simulink model "DiscreteAutogen_Controller"  (R2022a)
settings: Solver=FixedStepAuto  StartTime=0.0  StopTime=TsimTime  FixedStep=Ts  MaxStep=Tsim*100  RelTol=1e-5
undefined symbols (not defined in the file): A, Arpm, Avdc, b, Brpm, Bvdc, DiscIntNeverNeededParam, IbuckSaturation, IsatLimit, K, Ki_d, Ki_q, Kiv, Kiw, Kp_d, Kp_q, Kpv, Kpw, Krpm, Ktv, Ld, Lq, P, Rdc, Ts
libraries: simulink x4
settings Model: Creator=MasterGnome  LastModifiedBy=MasterGnome
settings SolverCC: ZeroCrossAlgorithm=Adaptive
settings DataIOCC: SaveOutput=off  SaveTime=off
settings OptimizationCC: DefaultParameterBehavior=Inlined  EnhancedBackFolding=on  PassReuseOutputArgsAs=Individual arguments  ZeroExternalMemoryAtStartup=off  ZeroInternalMemoryAtStartup=off  OptimizeBlockOrder=speed  DifferentSizesBufferReuse=on  OptimizationCustomize=off  EfficientTunableParamExpr=on
settings DebuggingCC: IgnoredZcDiagnostic=none  ParameterTunabilityLossMsg=error  UnconnectedInputMsg=warning  UnconnectedOutputMsg=warning  UnconnectedLineMsg=warning
settings HardwareCC: ProdBitPerPointer=32  ProdBitPerSizeT=32  ProdBitPerPtrDiffT=32  ProdWordSize=32  ProdHWDeviceType=Intel->x86-32 (Windows32)  TargetBitPerPointer=64  TargetBitPerSizeT=64  TargetBitPerPtrDiffT=64  TargetLargestAtomicFloat=Float  TargetIntDivRoundTo=Zero  TargetEndianess=LittleEndian  TargetWordSize=64  TargetHWDeviceType=Intel->x86-64 (Windows64)
settings SFSimCC: MATLABDynamicMemAlloc=off
settings RTWCC: SystemTargetFile=ert.tlc  GenCodeOnly=on  TemplateMakefile=ert_default_tmf  DLArmComputeVersion=19.05
settings CodeAppCC: ForceParamTrailComments=on  IgnoreCustomStorageClasses=off  OperatorAnnotations=on  SimulinkDataObjDesc=on  SFDataObjDesc=on  InsertBlockDesc=on
settings ERTTargetCC: TargetLangStandard=C99 (ISO)  GenerateSampleERTMain=on  InlinedParameterPlacement=NonHierarchical  ERTCustomFileTemplate=example_file_process.tlc

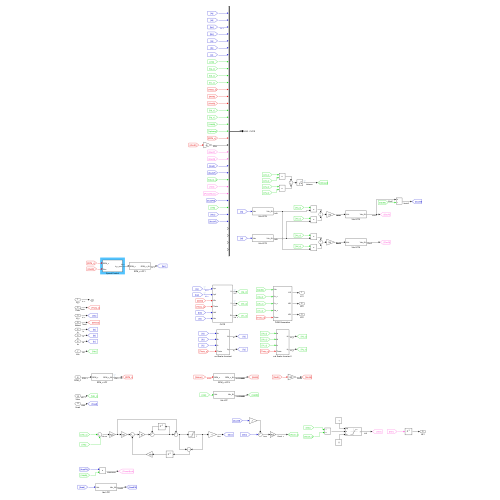
[thumbnail: Simulink's stored preview of the top-level diagram]
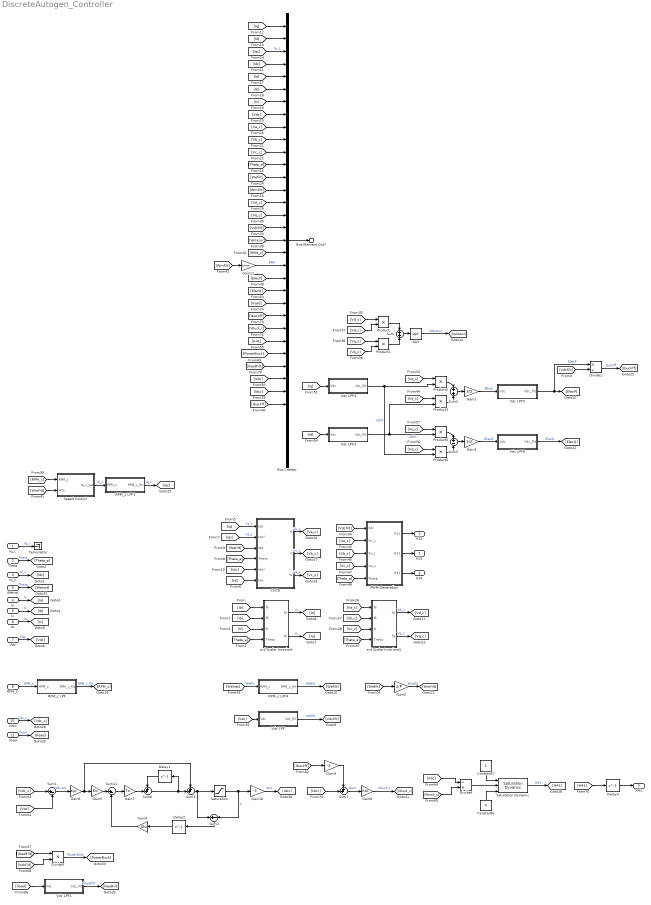
== system DiscreteAutogen_Controller ==
  Iq_c : Inport  OutDataTypeStr=double  PortDimensions=1
  Theta : Inport  Port=2  OutDataTypeStr=double  PortDimensions=1
  Id_c : Inport  Port=3  OutDataTypeStr=double  PortDimensions=1
  Iu : Inport  Port=4  OutDataTypeStr=double  PortDimensions=1
  Iv : Inport  Port=5  OutDataTypeStr=double  PortDimensions=1
  Iw : Inport  Port=6  OutDataTypeStr=double  PortDimensions=1
  Vdc : Inport  Port=7  OutDataTypeStr=double  PortDimensions=1
  RPM_C : Inport  Port=8  OutDataTypeStr=double  PortDimensions=1
  WeInst : Inport  Port=9  OutDataTypeStr=double  PortDimensions=1
  Vdcc : Inport  Port=10  OutDataTypeStr=double  PortDimensions=1
  Iload : Inport  Port=11  OutDataTypeStr=double  PortDimensions=1
  Bus Creator : BusCreator  Inputs=35
  CVCR : Subsystem
  Constant6 : Constant  Value=0
  Constant7 : Constant
  Delay1 : Delay  DelayLength=1  SampleTime=Ts
  Delay2 : Delay  DelayLength=1  SampleTime=Ts
  Delay3 : Delay  DelayLength=1  InitialCondition=0.1  SampleTime=Ts
  Divide1 : Product  Inputs=*/
  Divide3 : Product  Inputs=**
  Divide4 : Product  Inputs=/*
  Gain1 : Gain  Gain=3/2
  Gain11 : Gain  Gain=1/Krpm
  Gain16 : Gain  Gain=-1
  Gain2 : Gain  Gain=2/P
  Gain3 : Gain  Gain=3/2
  Gain4 : Gain  Gain=Ktv
  Gain5 : Gain  Gain=Kiv
  Gain6 : Gain  Gain=Kpv
  Gain7 : Gain  Gain=Ts
  Gain8 : Gain  Gain=Rdc
  Gain9 : Gain  Gain=-1
  PWM Generation : Subsystem
  Product{,1..3,5..6} (6 alike) : Product
  RPM_c LPF : Subsystem
  RPM_c LPF1 : Subsystem
  RPM_c LPF4 : Subsystem
  Saturation : Saturate  UpperLimit=0  LowerLimit=-IbuckSaturation
  Saturation Dynamic : simulink/Discontinuities/Saturation Dynamic  OutMin=[]  OutMax=[]  OutDataTypeStr=Inherit: Same as second input  OutDataType=fixdt(1, 16)  OutScaling=2^-10  DoSatur=off
  Speed Control : Subsystem
  Sqrt : Sqrt
  Sum : Sum  Inputs=+|+
  Sum1 : Sum  Inputs=|+-
  Sum11 : Sum  Inputs=|+-
  Sum2 : Sum  Inputs=+|+
  Sum3 : Sum  Inputs=++|
  Sum4 : Sum  Inputs=+|-
  Sum5 : Sum  Inputs=+|-
  Sum6 : Sum  Inputs=++|
  Sum7 : Sum  Inputs=++|
  Terminator : Terminator
  Vdc LPF : Subsystem
  Vdc LPF1 : Subsystem
  Vdc LPF3 : Subsystem
  Vdc LPF4 : Subsystem
  Vdc LPF5 : Subsystem
  Vdc LPF6 : Subsystem
  a-d Scalar Invariant : Subsystem
  a-d Scalar Invariant1 : Subsystem
  H11 : Outport  OutDataTypeStr=double  PortDimensions=1
  H21 : Outport  Port=2  OutDataTypeStr=double  PortDimensions=1
  H31 : Outport  Port=3  OutDataTypeStr=double  PortDimensions=1
  Bus Element Out7 : Outport  Port=4  PortName=LOG  Element=CVCR
  H41 : Outport  Port=5  OutDataTypeStr=double  PortDimensions=1
  wires:
  [Vc_c] -> PWM Generation/4(Vw_c)
  [Theta_e] -> PWM Generation/5(Theta)
  [Vb_c] -> PWM Generation/3(Vv_c)
  CVCR/2(V) -> [Vb_c]  "Vv_c"
  a-d Scalar Invariant/2(fq) -> [Iq]  "Iq"
  [Iq] -> CVCR/1(Iqe)  "Iq_c"
  CVCR/1(U) -> [Va_c]  "Vu_c"
  [Id] -> CVCR/6(Ide)
  CVCR/3(W) -> [Vc_c]  "Vw_c"
  [Vdcfilt] -> PWM Generation/1(Vdc)
  a-d Scalar Invariant/1(fd) -> [Id]  "Id"
  [Va_c] -> PWM Generation/2(Vu_c)
  PWM Generation/1(H11) -> H11/1
  PWM Generation/2(H21) -> H21/1
  PWM Generation/3(H31) -> H31/1
  [Wefilt] -> CVCR/3(We)
  [Theta_e] -> CVCR/4(Theta)
  [Theta_e] -> a-d Scalar Invariant/4(Theta)
  [Ib] -> a-d Scalar Invariant/2(fb)
  [Ic] -> a-d Scalar Invariant/3(fc)
  [Ia] -> a-d Scalar Invariant/1(fa)
  Iu/1 -> [Ia]  "Iu"
  Iv/1 -> [Ib]  "Iv"
  Iw/1 -> [Ic]  "Iw"
  Vdc/1 -> [Vdc]  "Vdc"
  [WeInst] -> RPM_c LPF4/1(RPM_c)  "Wefilt"
  Id_c/1 -> [Idc]  "Id_c"
  [Iqc] -> CVCR/2(Iqe*)  "Id_c"
  [Idc] -> CVCR/5(Ide*)
  Bus Creator/1 -> Bus Element Out7/1
  [Iq] -> Bus Creator/1
  [Id] -> Bus Creator/2
  [Iqc] -> Bus Creator/3  "Iq_c"
  [Idc] -> Bus Creator/4
  [Ia] -> Bus Creator/5
  [Ib] -> Bus Creator/6
  [Ic] -> Bus Creator/7
  [Vdc] -> Bus Creator/8
  [Va_c] -> Bus Creator/9
  [Vb_c] -> Bus Creator/10
  [Vc_c] -> Bus Creator/11
  [Theta_e] -> Bus Creator/12
  [Wefilt] -> Bus Creator/13
  [Theta_e] -> a-d Scalar Invariant1/4(Theta)
  [Va_c] -> a-d Scalar Invariant1/1(fa)
  [Vb_c] -> a-d Scalar Invariant1/2(fb)
  [Vc_c] -> a-d Scalar Invariant1/3(fc)
  a-d Scalar Invariant1/1(fd) -> [Vd_c]  "Vd_c"
  a-d Scalar Invariant1/2(fq) -> [Vq_c]  "Vq_c"
  [Vq_c] -> Bus Creator/16
  [Vd_c] -> Bus Creator/15
  [Wefilt] -> Gain2/1
  [Wmfilt] -> Bus Creator/14
  [Vdc] -> Vdc LPF/1(Vdc)
  Vdc LPF/1(Vdc_filt) -> [Vdcfilt]  "Vdcfilt"
  [Vdcfilt] -> Bus Creator/17
  [Vd_c] -> Product/1
  [Vd_c] -> Product/2
  [Vq_c] -> Product1/1
  [Vq_c] -> Product1/2
  Product/1 -> Sum/1
  Product1/1 -> Sum/2
  Sum/1 -> Sqrt/1
  Sqrt/1 -> [Vphasor]  "Vphasor"
  [Vphasor] -> Bus Creator/18
  Theta/1 -> [Theta_e]  "Theta"
  [Wmfilt] -> Speed Control/2(Wm)
  [RPM_c] -> Bus Creator/19
  Gain11/1 -> Bus Creator/20  "RPM"
  [Wmfilt] -> Gain11/1
  Speed Control/1(Iq_c_sat) -> RPM_c LPF1/1(RPM_c)  "Iq_c"
  [Vd_c] -> Product3/1
  Gain3/1 -> Vdc LPF6/1(Vdc)  "ElecQ"
  Product5/1 -> Sum5/1
  Sum2/1 -> Gain1/1
  Product3/1 -> Sum2/2
  Product2/1 -> Sum2/1
  Sum5/1 -> Gain3/1
  [Vq_c] -> Product2/1
  Product6/1 -> Sum5/2
  [Vd_c] -> Product6/1
  [Vq_c] -> Product5/1
  [ElecP] -> Bus Creator/21
  [ElecQ] -> Bus Creator/22
  RPM_C/1 -> RPM_c LPF/1(RPM_c)  "RPM_c"
  [RPM_c] -> Speed Control/1(RPM_c)
  RPM_c LPF/1(RPM_c_filt) -> [RPM_c]  "RPM_c_filt"
  Iq_c/1 -> Terminator/1  "Iq_c"
  RPM_c LPF1/1(RPM_c_filt) -> [Iqc]  "Iq_c"
  Gain2/1 -> [Wmfilt]  "Wmfilt"
  WeInst/1 -> [WeInst]  "Theta"
  RPM_c LPF4/1(RPM_c_filt) -> [Wefilt]  "Wefilt"
  Divide1/1 -> [Ibuckff]  "Ibuckff"
  Gain1/1 -> Vdc LPF5/1(Vdc)  "PElec"
  [Vdcfilt] -> Divide1/2
  Vdc LPF5/1(Vdc_filt) -> Divide1/1, [ElecP]  "ElecP"
  Vdc LPF6/1(Vdc_filt) -> [ElecQ]  "ElecQ"
  [Id] -> Vdc LPF3/1(Vdc)
  Vdc LPF3/1(Vdc_filt) -> Product3/2, Product5/2  "Idfilt"
  [Iq] -> Vdc LPF4/1(Vdc)
  Vdc LPF4/1(Vdc_filt) -> Product6/2, Product2/2  "Iqfilt"
  Sum4/1 -> Delay2/1
  [Vdcfilt] -> Divide3/2
  Delay2/1 -> Gain4/1
  Gain7/1 -> Sum6/2
  Vdc LPF1/1(Vdc_filt) -> [IloadFilt]  "Iloadfilt"
  Delay1/1 -> Sum6/1
  Gain16/1 -> [Idcc]  "Idcc"
  Sum6/1 -> Sum3/2, Delay1/1
  Constant6/1 -> Saturation Dynamic/3
  [Vbuck_c] -> Divide4/2
  Constant7/1 -> Saturation Dynamic/1
  [Vdc] -> Divide4/1
  [Vdc] -> Sum1/2
  Divide3/1 -> [PowerBuck]  "PowerBuck"
  [Iload] -> Vdc LPF1/1(Vdc)
  Saturation/1 -> Gain16/1, Sum4/2  "I*"
  [Vdc_c] -> Sum1/1
  Sum1/1 -> Gain6/1  "Vdc err"
  [H41] -> Delay3/1
  [Idcc] -> Sum7/2
  Sum7/1 -> Gain8/1  "Isum"
  Sum3/1 -> Sum4/1, Saturation/1
  Gain5/1 -> Sum11/1
  Divide4/1 -> Saturation Dynamic/2
  Sum11/1 -> Gain7/1
  Gain8/1 -> [Vbuck_c]  "Vbuck_c"
  [IloadFilt] -> Divide3/1
  Gain4/1 -> Sum11/2
  Vdcc/1 -> [Vdc_c]  "Vdc_c"
  Iload/1 -> [Iload]  "Iload"
  Saturation Dynamic/1 -> [H41]  "H41"
  Gain6/1 -> Gain5/1, Sum3/1
  [Vbuck_c] -> Bus Creator/25
  [Iload] -> Bus Creator/23
  [Ibuckff] -> Bus Creator/24
  [PowerBuck] -> Bus Creator/27
  [IloadFilt] -> Bus Creator/28
  [H41] -> Bus Creator/26
  [Ibuckff] -> Gain9/1
  Gain9/1 -> Sum7/1
  Delay3/1 -> H41/1
  [Vdc] -> Bus Creator/29
  [Idcc] -> Bus Creator/30
  [Ibuckff] -> Bus Creator/31

== system DiscreteAutogen_Controller/CVCR ==
  Iqe : Inport
  Iqe* : Inport  Port=2
  We : Inport  Port=3
  Theta : Inport  Port=4
  Ide* : Inport  Port=5
  Ide : Inport  Port=6
  "CVCR - Complex " : Subsystem  Commented=on
  CVCR Tustin Xcouple : Subsystem  Commented=on
  PI Tustin : Subsystem  Commented=on
  PI Zoh Parallel Xcouple : Subsystem  Commented=on
  PI Zoh Parallel1 : Subsystem  Commented=on
  PI Zoh Series : Subsystem  Commented=on
  PI Zoh Series Xcouple : Subsystem
  d-a Scalar Invariant : Subsystem
  q-a Scalar Invariant : Subsystem  Commented=on
  U : Outport
  V : Outport  Port=2
  W : Outport  Port=3
  wires:
  PI Zoh Series Xcouple/2(Vde) -> d-a Scalar Invariant/2(fd)  "Vd*"
  PI Zoh Series Xcouple/1(Vqe) -> d-a Scalar Invariant/1(fq)  "Vq*"
  Ide/1 -> PI Zoh Series Xcouple/5(Id)
  Ide*/1 -> PI Zoh Series Xcouple/4(Id_c)
  Iqe*/1 -> PI Zoh Series Xcouple/2(Iq_c)
  Iqe/1 -> PI Zoh Series Xcouple/1(Iq)
  d-a Scalar Invariant/2(b) -> V/1
  d-a Scalar Invariant/1(a) -> U/1
  Theta/1 -> d-a Scalar Invariant/3(theta)
  We/1 -> PI Zoh Series Xcouple/3(We)
  d-a Scalar Invariant/3(c) -> W/1

== system DiscreteAutogen_Controller/PWM Generation ==
  Vdc : Inport
  Vu_c : Inport  Port=2
  Vv_c : Inport  Port=3
  Vw_c : Inport  Port=4
  Theta : Inport  Port=5
  Duty Cycle Calc : Subsystem
  Modulation : Subsystem
  H11 : Outport
  H21 : Outport  Port=2
  H31 : Outport  Port=3
  wires:
  Vw_c/1 -> Modulation/4(Vc_c)
  Theta/1 -> Modulation/5(Theta)
  Vv_c/1 -> Modulation/3(Vb_c)
  Vu_c/1 -> Modulation/2(Va_c)
  Vdc/1 -> Modulation/1(Vdc), [Vdc]
  Duty Cycle Calc/3(H31) -> H31/1
  [Vdc] -> Duty Cycle Calc/1(Vdc)
  [Va_mod] -> Duty Cycle Calc/2(Va_mod)
  Modulation/3(Vc_mod) -> [Vc_mod]
  [Vc_mod] -> Duty Cycle Calc/4(Vc_mod)
  Duty Cycle Calc/2(H21) -> H21/1
  [Vb_mod] -> Duty Cycle Calc/3(Vb_mod)
  Duty Cycle Calc/1(H11) -> H11/1
  Modulation/2(Vb_mod) -> [Vb_mod]
  Modulation/1(Va_mod) -> [Va_mod]

== system DiscreteAutogen_Controller/RPM_c LPF ==
  RPM_c : Inport
  Delay2 : Delay  DelayLength=1  InitialCondition=0  SampleTime=Ts
  Gain1 : Gain  Gain=Brpm
  Gain3 : Gain  Gain=Arpm
  Sum2 : Sum  Inputs=|++
  RPM_c_filt : Outport
  wires:
  RPM_c/1 -> Gain1/1
  Delay2/1 -> RPM_c_filt/1, Gain3/1
  Sum2/1 -> Delay2/1
  Gain1/1 -> Sum2/1
  Gain3/1 -> Sum2/2

== system DiscreteAutogen_Controller/RPM_c LPF1 ==
  RPM_c : Inport
  Delay2 : Delay  DelayLength=1  InitialCondition=0  SampleTime=Ts
  Gain1 : Gain  Gain=Brpm
  Gain3 : Gain  Gain=Arpm
  Sum2 : Sum  Inputs=|++
  RPM_c_filt : Outport
  wires:
  RPM_c/1 -> Gain1/1
  Delay2/1 -> RPM_c_filt/1, Gain3/1
  Sum2/1 -> Delay2/1
  Gain1/1 -> Sum2/1
  Gain3/1 -> Sum2/2

== system DiscreteAutogen_Controller/RPM_c LPF4 ==
  RPM_c : Inport
  Delay2 : Delay  DelayLength=1  InitialCondition=0  SampleTime=Ts
  Gain1 : Gain  Gain=Brpm
  Gain3 : Gain  Gain=Arpm
  Sum2 : Sum  Inputs=|++
  RPM_c_filt : Outport
  wires:
  RPM_c/1 -> Gain1/1
  Delay2/1 -> RPM_c_filt/1, Gain3/1
  Sum2/1 -> Delay2/1
  Gain1/1 -> Sum2/1
  Gain3/1 -> Sum2/2

== system DiscreteAutogen_Controller/Speed Control ==
  RPM_c : Inport
  Wm : Inport  Port=2
  Delay1 : Delay  DelayLength=1  SampleTime=Ts
  Delay3 : Delay  DelayLength=1  SampleTime=Ts
  Gain11 : Gain  Gain=Krpm
  Gain4 : Gain  Gain=Kpw
  Gain5 : Gain  Gain=Ts
  Gain6 : Gain  Gain=Kiw
  Kt1 : Gain
  Saturation2 : Saturate  UpperLimit=IsatLimit  LowerLimit=-IsatLimit
  Sum11 : Sum  Inputs=+|-
  Sum12 : Sum  Inputs=|+-
  Sum6 : Sum  Inputs=++|
  Sum7 : Sum  Inputs=+++
  Sum9 : Sum  Inputs=|+-
  Iq_c_sat : Outport
  wires:
  Sum7/1 -> Saturation2/1, Sum11/1  "Iq_c_z"
  Sum12/1 -> Gain5/1
  Sum6/1 -> Sum7/2, Delay1/1
  Sum11/1 -> Delay3/1
  Sum9/1 -> Gain4/1
  Gain6/1 -> Sum12/1
  Gain5/1 -> Sum6/2
  Delay1/1 -> Sum6/1
  RPM_c/1 -> Gain11/1
  Gain11/1 -> Sum9/1  "Wm_c"
  Wm/1 -> Sum9/2
  Saturation2/1 -> Iq_c_sat/1, Sum11/2
  Delay3/1 -> Kt1/1
  Kt1/1 -> Sum12/2
  Gain4/1 -> Sum7/1, Gain6/1

== system DiscreteAutogen_Controller/Vdc LPF ==
  Vdc : Inport
  Delay2 : Delay  DelayLength=1  InitialCondition=0  SampleTime=Ts
  Gain1 : Gain  Gain=Bvdc
  Gain3 : Gain  Gain=Avdc
  Sum2 : Sum  Inputs=|++
  Vdc_filt : Outport
  wires:
  Vdc/1 -> Gain1/1
  Delay2/1 -> Vdc_filt/1, Gain3/1
  Sum2/1 -> Delay2/1
  Gain1/1 -> Sum2/1
  Gain3/1 -> Sum2/2

== system DiscreteAutogen_Controller/Vdc LPF1 ==
  Vdc : Inport
  Delay2 : Delay  DelayLength=1  InitialCondition=1  SampleTime=Ts
  Gain1 : Gain  Gain=Bvdc
  Gain3 : Gain  Gain=Avdc
  Sum2 : Sum  Inputs=|++
  Vdc_filt : Outport
  wires:
  Vdc/1 -> Gain1/1
  Delay2/1 -> Vdc_filt/1, Gain3/1
  Sum2/1 -> Delay2/1
  Gain1/1 -> Sum2/1
  Gain3/1 -> Sum2/2

== system DiscreteAutogen_Controller/Vdc LPF3 ==
  Vdc : Inport
  Delay2 : Delay  DelayLength=1  InitialCondition=0  SampleTime=Ts
  Gain1 : Gain  Gain=Bvdc
  Gain3 : Gain  Gain=Avdc
  Sum2 : Sum  Inputs=|++
  Vdc_filt : Outport
  wires:
  Vdc/1 -> Gain1/1
  Delay2/1 -> Vdc_filt/1, Gain3/1
  Sum2/1 -> Delay2/1
  Gain1/1 -> Sum2/1
  Gain3/1 -> Sum2/2

== system DiscreteAutogen_Controller/Vdc LPF4 ==
  Vdc : Inport
  Delay2 : Delay  DelayLength=1  InitialCondition=0  SampleTime=Ts
  Gain1 : Gain  Gain=Bvdc
  Gain3 : Gain  Gain=Avdc
  Sum2 : Sum  Inputs=|++
  Vdc_filt : Outport
  wires:
  Vdc/1 -> Gain1/1
  Delay2/1 -> Vdc_filt/1, Gain3/1
  Sum2/1 -> Delay2/1
  Gain1/1 -> Sum2/1
  Gain3/1 -> Sum2/2

== system DiscreteAutogen_Controller/Vdc LPF5 ==
  Vdc : Inport
  Delay2 : Delay  DelayLength=1  InitialCondition=0  SampleTime=Ts
  Gain1 : Gain  Gain=Bvdc
  Gain3 : Gain  Gain=Avdc
  Sum2 : Sum  Inputs=|++
  Vdc_filt : Outport
  wires:
  Vdc/1 -> Gain1/1
  Delay2/1 -> Vdc_filt/1, Gain3/1
  Sum2/1 -> Delay2/1
  Gain1/1 -> Sum2/1
  Gain3/1 -> Sum2/2

== system DiscreteAutogen_Controller/Vdc LPF6 ==
  Vdc : Inport
  Delay2 : Delay  DelayLength=1  InitialCondition=0  SampleTime=Ts
  Gain1 : Gain  Gain=Bvdc
  Gain3 : Gain  Gain=Avdc
  Sum2 : Sum  Inputs=|++
  Vdc_filt : Outport
  wires:
  Vdc/1 -> Gain1/1
  Delay2/1 -> Vdc_filt/1, Gain3/1
  Sum2/1 -> Delay2/1
  Gain1/1 -> Sum2/1
  Gain3/1 -> Sum2/2

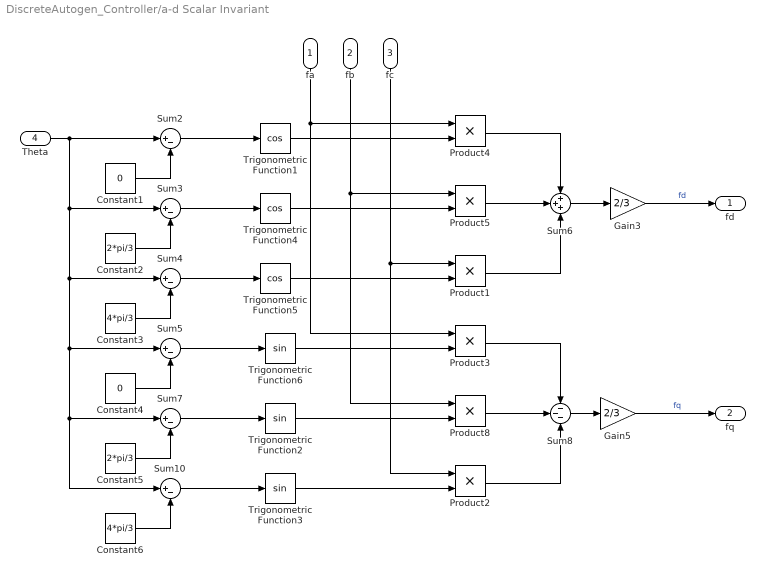
== system DiscreteAutogen_Controller/a-d Scalar Invariant ==
  fa : Inport
  fb : Inport  Port=2
  fc : Inport  Port=3
  Theta : Inport  Port=4
  Constant1 : Constant  Value=0
  Constant2 : Constant  Value=2*pi/3
  Constant3 : Constant  Value=4*pi/3
  Constant4 : Constant  Value=0
  Constant5 : Constant  Value=2*pi/3
  Constant6 : Constant  Value=4*pi/3
  Gain3 : Gain  Gain=2/3
  Gain5 : Gain  Gain=2/3
  Product{1..5,8} (6 alike) : Product
  Sum{2..5,7,10} (6 alike) : Sum  Inputs=|+-
  Sum6 : Sum  Inputs=+++
  Sum8 : Sum  Inputs=---
  Trigonometric Function1 : Trigonometry  Operator=cos
  Trigonometric Function2 : Trigonometry
  Trigonometric Function3 : Trigonometry
  Trigonometric Function4 : Trigonometry  Operator=cos
  Trigonometric Function5 : Trigonometry  Operator=cos
  Trigonometric Function6 : Trigonometry
  fd : Outport
  fq : Outport  Port=2
  wires:
  Product1/1 -> Sum6/3
  fc/1 -> Product2/1, Product1/1
  Sum4/1 -> Trigonometric Function5/1
  Constant5/1 -> Sum7/2
  Trigonometric Function4/1 -> Product5/2
  Sum7/1 -> Trigonometric Function2/1
  Constant6/1 -> Sum10/2
  Trigonometric Function3/1 -> Product2/2
  Theta/1 -> Sum10/1, Sum7/1, Sum5/1, Sum4/1, Sum3/1, Sum2/1
  Sum10/1 -> Trigonometric Function3/1
  Sum5/1 -> Trigonometric Function6/1
  Product2/1 -> Sum8/3
  Trigonometric Function2/1 -> Product8/2
  Product3/1 -> Sum8/1
  Constant3/1 -> Sum4/2
  Trigonometric Function1/1 -> Product4/2
  Product8/1 -> Sum8/2
  Trigonometric Function5/1 -> Product1/2
  Constant2/1 -> Sum3/2
  Sum3/1 -> Trigonometric Function4/1
  Sum8/1 -> Gain5/1
  Constant4/1 -> Sum5/2
  Constant1/1 -> Sum2/2
  Sum2/1 -> Trigonometric Function1/1
  fa/1 -> Product4/1, Product3/1
  Gain3/1 -> fd/1  "fd"
  Sum6/1 -> Gain3/1
  Trigonometric Function6/1 -> Product3/2
  Product4/1 -> Sum6/1
  Gain5/1 -> fq/1  "fq"
  fb/1 -> Product5/1, Product8/1
  Product5/1 -> Sum6/2

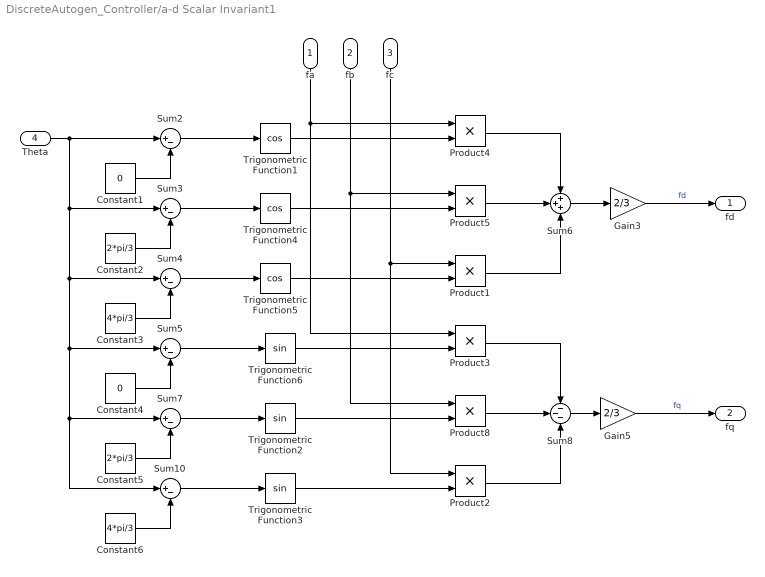
== system DiscreteAutogen_Controller/a-d Scalar Invariant1 ==
  fa : Inport
  fb : Inport  Port=2
  fc : Inport  Port=3
  Theta : Inport  Port=4
  Constant1 : Constant  Value=0
  Constant2 : Constant  Value=2*pi/3
  Constant3 : Constant  Value=4*pi/3
  Constant4 : Constant  Value=0
  Constant5 : Constant  Value=2*pi/3
  Constant6 : Constant  Value=4*pi/3
  Gain3 : Gain  Gain=2/3
  Gain5 : Gain  Gain=2/3
  Product{1..5,8} (6 alike) : Product
  Sum{2..5,7,10} (6 alike) : Sum  Inputs=|+-
  Sum6 : Sum  Inputs=+++
  Sum8 : Sum  Inputs=---
  Trigonometric Function1 : Trigonometry  Operator=cos
  Trigonometric Function2 : Trigonometry
  Trigonometric Function3 : Trigonometry
  Trigonometric Function4 : Trigonometry  Operator=cos
  Trigonometric Function5 : Trigonometry  Operator=cos
  Trigonometric Function6 : Trigonometry
  fd : Outport
  fq : Outport  Port=2
  wires:
  Product1/1 -> Sum6/3
  fc/1 -> Product2/1, Product1/1
  Sum4/1 -> Trigonometric Function5/1
  Constant5/1 -> Sum7/2
  Trigonometric Function4/1 -> Product5/2
  Sum7/1 -> Trigonometric Function2/1
  Constant6/1 -> Sum10/2
  Trigonometric Function3/1 -> Product2/2
  Theta/1 -> Sum10/1, Sum7/1, Sum5/1, Sum4/1, Sum3/1, Sum2/1
  Sum10/1 -> Trigonometric Function3/1
  Sum5/1 -> Trigonometric Function6/1
  Product2/1 -> Sum8/3
  Trigonometric Function2/1 -> Product8/2
  Product3/1 -> Sum8/1
  Constant3/1 -> Sum4/2
  Trigonometric Function1/1 -> Product4/2
  Product8/1 -> Sum8/2
  Trigonometric Function5/1 -> Product1/2
  Constant2/1 -> Sum3/2
  Sum3/1 -> Trigonometric Function4/1
  Sum8/1 -> Gain5/1
  Constant4/1 -> Sum5/2
  Constant1/1 -> Sum2/2
  Sum2/1 -> Trigonometric Function1/1
  fa/1 -> Product4/1, Product3/1
  Gain3/1 -> fd/1  "fd"
  Sum6/1 -> Gain3/1
  Trigonometric Function6/1 -> Product3/2
  Product4/1 -> Sum6/1
  Gain5/1 -> fq/1  "fq"
  fb/1 -> Product5/1, Product8/1
  Product5/1 -> Sum6/2

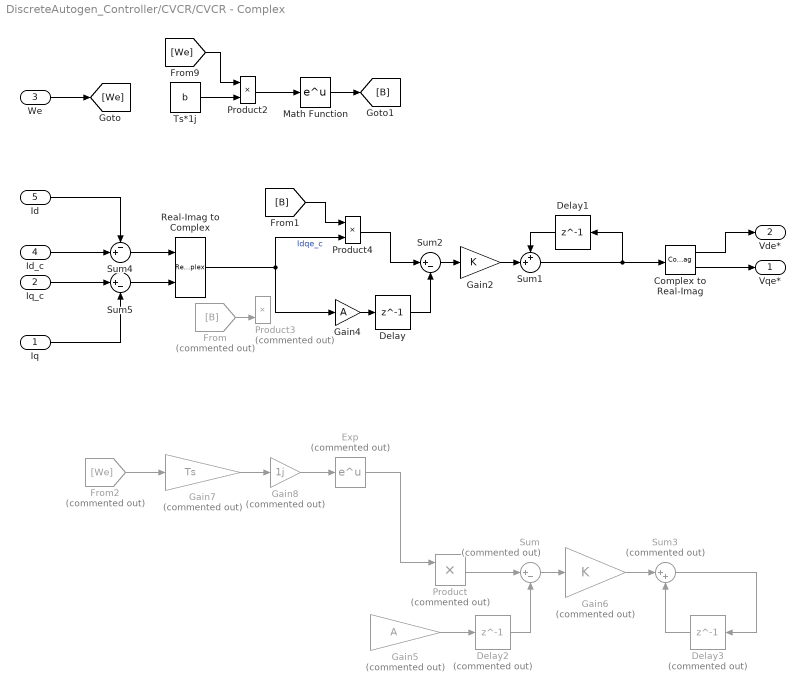
== system DiscreteAutogen_Controller/CVCR/CVCR - Complex  ==
  Iq : Inport
  Iq_c : Inport  Port=2
  We : Inport  Port=3
  Id_c : Inport  Port=4
  Id : Inport  Port=5
  Complex to Real-Imag : ComplexToRealImag
  Delay : Delay  DelayLength=1
  Delay1 : Delay  DelayLength=1
  Delay2 : Delay  Commented=on  DelayLength=1
  Delay3 : Delay  Commented=on  DelayLength=1
  Exp : Math  Commented=on
  From : From  Commented=on  GotoTag=B
  From2 : From  Commented=on  GotoTag=We
  Gain2 : Gain  Gain=K
  Gain4 : Gain  Gain=A
  Gain5 : Gain  Commented=on  Gain=A
  Gain6 : Gain  Commented=on  Gain=K
  Gain7 : Gain  Commented=on  Gain=Ts
  Gain8 : Gain  Commented=on  Gain=1j
  Math Function : Math
  Product : Product  Commented=on
  Product2 : Product
  Product3 : Product  Commented=on
  Product4 : Product
  Real-Imag to Complex : RealImagToComplex
  Sum : Sum  Commented=on  Inputs=|+-
  Sum1 : Sum  Inputs=++|
  Sum2 : Sum  Inputs=|+-
  Sum3 : Sum  Commented=on  Inputs=|++
  Sum4 : Sum  Inputs=-+|
  Sum5 : Sum  Inputs=|+-
  Ts*1j : Constant  Value=b
  Vqe* : Outport
  Vde* : Outport  Port=2
  wires:
  Sum5/1 -> Real-Imag to Complex/2
  Sum4/1 -> Real-Imag to Complex/1
  Id_c/1 -> Sum4/2
  Id/1 -> Sum4/1
  Iq_c/1 -> Sum5/1
  Iq/1 -> Sum5/2
  Complex to Real-Imag/2 -> Vqe*/1
  Complex to Real-Imag/1 -> Vde*/1
  We/1 -> [We]
  [We] -> Product2/1
  Math Function/1 -> [B]
  From/1 -> Product3/2
  Gain4/1 -> Delay/1
  Delay/1 -> Sum2/2
  Delay1/1 -> Sum1/1
  Product2/1 -> Math Function/1
  Sum2/1 -> Gain2/1
  Gain2/1 -> Sum1/2
  Sum1/1 -> Complex to Real-Imag/1, Delay1/1
  [B] -> Product4/1
  Product4/1 -> Sum2/1
  From2/1 -> Gain7/1
  Sum/1 -> Gain6/1
  Sum3/1 -> Delay3/1
  Gain5/1 -> Delay2/1
  Exp/1 -> Product/1
  Delay2/1 -> Sum/2
  Gain6/1 -> Sum3/1
  Delay3/1 -> Sum3/2
  Product/1 -> Sum/1
  Gain7/1 -> Gain8/1
  Gain8/1 -> Exp/1
  ? -> Gain5/1, Product/2
  Ts*1j/1 -> Product2/2
  Real-Imag to Complex/1 -> Product4/2, Gain4/1  "Idqe_c"

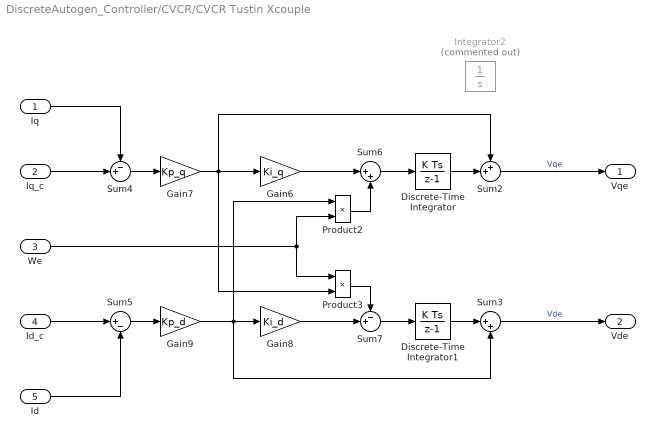
== system DiscreteAutogen_Controller/CVCR/CVCR Tustin Xcouple ==
  Iq : Inport
  Iq_c : Inport  Port=2
  We : Inport  Port=3
  Id_c : Inport  Port=4
  Id : Inport  Port=5
  Discrete-Time Integrator : DiscreteIntegrator  SampleTime=Ts  ICPrevOutput=DiscIntNeverNeededParam  ICPrevScaledInput=DiscIntNeverNeededParam
  Discrete-Time Integrator1 : DiscreteIntegrator  SampleTime=Ts  ICPrevOutput=DiscIntNeverNeededParam  ICPrevScaledInput=DiscIntNeverNeededParam
  Gain6 : Gain  Gain=Ki_q
  Gain7 : Gain  Gain=Kp_q
  Gain8 : Gain  Gain=Ki_d
  Gain9 : Gain  Gain=Kp_d
  Integrator2 : Integrator  Commented=on
  Product2 : Product
  Product3 : Product
  Sum2 : Sum  Inputs=++|
  Sum3 : Sum  Inputs=|++
  Sum4 : Sum  Inputs=-+|
  Sum5 : Sum  Inputs=|+-
  Sum6 : Sum  Inputs=|++
  Sum7 : Sum  Inputs=-+|
  Vqe : Outport
  Vde : Outport  Port=2
  wires:
  Sum3/1 -> Vde/1  "Vde"
  Id_c/1 -> Sum5/1
  Sum2/1 -> Vqe/1  "Vqe"
  Iq/1 -> Sum4/1
  Gain6/1 -> Sum6/1
  Sum7/1 -> Discrete-Time Integrator1/1
  Sum4/1 -> Gain7/1
  Gain8/1 -> Sum7/2
  Discrete-Time Integrator/1 -> Sum2/2
  Iq_c/1 -> Sum4/2
  Id/1 -> Sum5/2
  Sum6/1 -> Discrete-Time Integrator/1
  Product3/1 -> Sum7/1
  Gain7/1 -> Product3/2, Sum2/1, Gain6/1
  Product2/1 -> Sum6/2
  Discrete-Time Integrator1/1 -> Sum3/1
  Sum5/1 -> Gain9/1
  Gain9/1 -> Sum3/2, Gain8/1, Product2/1
  We/1 -> Product3/1, Product2/2

== system DiscreteAutogen_Controller/CVCR/PI Tustin ==
  Iq : Inport
  Iq_c : Inport  Port=2
  We : Inport  Port=3
  Id_c : Inport  Port=4
  Id : Inport  Port=5
  Discrete-Time Integrator : DiscreteIntegrator  SampleTime=Ts  ICPrevOutput=DiscIntNeverNeededParam  ICPrevScaledInput=DiscIntNeverNeededParam
  Discrete-Time Integrator1 : DiscreteIntegrator  SampleTime=Ts  ICPrevOutput=DiscIntNeverNeededParam  ICPrevScaledInput=DiscIntNeverNeededParam
  Gain6 : Gain  Gain=Ki_q
  Gain7 : Gain  Gain=Kp_q
  Gain8 : Gain  Gain=Ki_d
  Gain9 : Gain  Gain=Kp_d
  Sum2 : Sum  Inputs=++|
  Sum3 : Sum  Inputs=|++
  Sum4 : Sum  Inputs=-+|
  Sum5 : Sum  Inputs=|+-
  Sum6 : Sum  Inputs=|++
  Sum7 : Sum  Inputs=-+|
  Vqe : Outport
  Vde : Outport  Port=2
  wires:
  Sum3/1 -> Vde/1  "Vde"
  Id_c/1 -> Sum5/1
  Sum2/1 -> Vqe/1  "Vqe"
  Iq/1 -> Sum4/1
  Gain6/1 -> Sum6/1
  Sum7/1 -> Discrete-Time Integrator1/1
  Sum4/1 -> Gain7/1
  Gain8/1 -> Sum7/2
  Discrete-Time Integrator/1 -> Sum2/2
  Iq_c/1 -> Sum4/2
  Id/1 -> Sum5/2
  Sum6/1 -> Discrete-Time Integrator/1
  Gain7/1 -> Sum2/1, Gain6/1
  Discrete-Time Integrator1/1 -> Sum3/1
  Sum5/1 -> Gain9/1
  Gain9/1 -> Sum3/2, Gain8/1

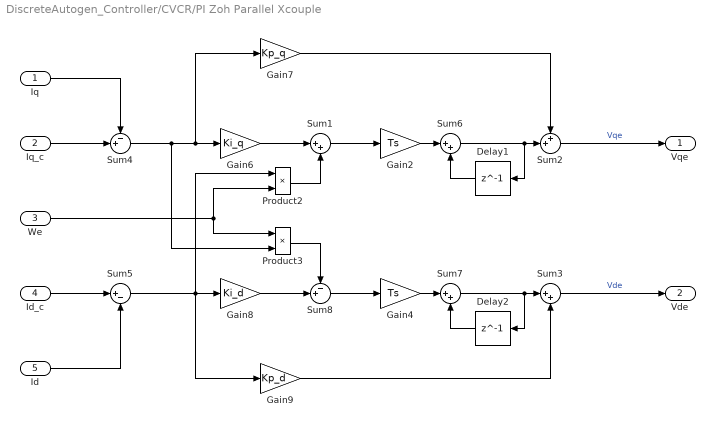
== system DiscreteAutogen_Controller/CVCR/PI Zoh Parallel Xcouple ==
  Iq : Inport
  Iq_c : Inport  Port=2
  We : Inport  Port=3
  Id_c : Inport  Port=4
  Id : Inport  Port=5
  Delay1 : Delay  DelayLength=1  SampleTime=Ts
  Delay2 : Delay  DelayLength=1  SampleTime=Ts
  Gain2 : Gain  Gain=Ts
  Gain4 : Gain  Gain=Ts
  Gain6 : Gain  Gain=Ki_q
  Gain7 : Gain  Gain=Kp_q
  Gain8 : Gain  Gain=Ki_d
  Gain9 : Gain  Gain=Kp_d
  Product2 : Product
  Product3 : Product
  Sum{1,3,6..7} (4 alike) : Sum  Inputs=|++
  Sum2 : Sum  Inputs=++|
  Sum4 : Sum  Inputs=-+|
  Sum5 : Sum  Inputs=|+-
  Sum8 : Sum  Inputs=-+|
  Vqe : Outport
  Vde : Outport  Port=2
  wires:
  Sum3/1 -> Vde/1  "Vde"
  Id_c/1 -> Sum5/1
  Sum2/1 -> Vqe/1  "Vqe"
  Iq/1 -> Sum4/1
  Gain6/1 -> Sum1/1
  Sum6/1 -> Delay1/1, Sum2/2
  Iq_c/1 -> Sum4/2
  Id/1 -> Sum5/2
  Gain7/1 -> Sum2/1
  Gain9/1 -> Sum3/2
  Gain2/1 -> Sum6/1
  Delay1/1 -> Sum6/2
  Gain4/1 -> Sum7/1
  Delay2/1 -> Sum7/2
  Sum7/1 -> Sum3/1, Delay2/1
  Sum4/1 -> Product3/2, Gain6/1, Gain7/1
  Product3/1 -> Sum8/1
  Sum5/1 -> Gain9/1, Product2/1, Gain8/1
  Product2/1 -> Sum1/2
  We/1 -> Product3/1, Product2/2
  Sum1/1 -> Gain2/1
  Gain8/1 -> Sum8/2
  Sum8/1 -> Gain4/1

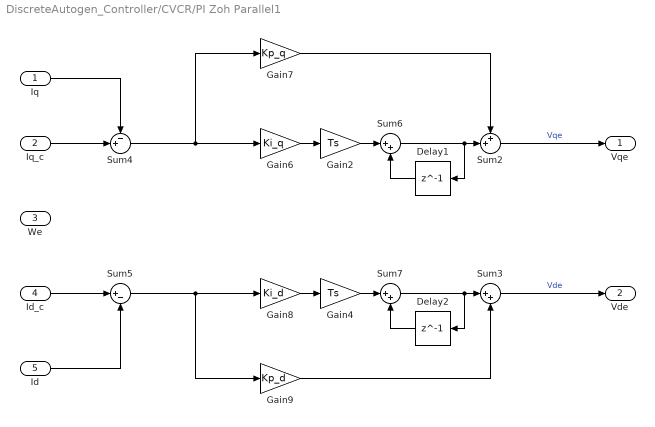
== system DiscreteAutogen_Controller/CVCR/PI Zoh Parallel1 ==
  Iq : Inport
  Iq_c : Inport  Port=2
  We : Inport  Port=3
  Id_c : Inport  Port=4
  Id : Inport  Port=5
  Delay1 : Delay  DelayLength=1  SampleTime=Ts
  Delay2 : Delay  DelayLength=1  SampleTime=Ts
  Gain2 : Gain  Gain=Ts
  Gain4 : Gain  Gain=Ts
  Gain6 : Gain  Gain=Ki_q
  Gain7 : Gain  Gain=Kp_q
  Gain8 : Gain  Gain=Ki_d
  Gain9 : Gain  Gain=Kp_d
  Sum2 : Sum  Inputs=++|
  Sum3 : Sum  Inputs=|++
  Sum4 : Sum  Inputs=-+|
  Sum5 : Sum  Inputs=|+-
  Sum6 : Sum  Inputs=|++
  Sum7 : Sum  Inputs=|++
  Vqe : Outport
  Vde : Outport  Port=2
  wires:
  Sum3/1 -> Vde/1  "Vde"
  Id_c/1 -> Sum5/1
  Sum2/1 -> Vqe/1  "Vqe"
  Iq/1 -> Sum4/1
  Gain6/1 -> Gain2/1
  Sum4/1 -> Gain6/1, Gain7/1
  Sum6/1 -> Delay1/1, Sum2/2
  Iq_c/1 -> Sum4/2
  Id/1 -> Sum5/2
  Gain7/1 -> Sum2/1
  Sum5/1 -> Gain8/1, Gain9/1
  Gain9/1 -> Sum3/2
  Gain2/1 -> Sum6/1
  Delay1/1 -> Sum6/2
  Gain4/1 -> Sum7/1
  Delay2/1 -> Sum7/2
  Sum7/1 -> Sum3/1, Delay2/1
  Gain8/1 -> Gain4/1

== system DiscreteAutogen_Controller/CVCR/PI Zoh Series ==
  Iq : Inport
  Iq_c : Inport  Port=2
  We : Inport  Port=3
  Id_c : Inport  Port=4
  Id : Inport  Port=5
  Delay1 : Delay  DelayLength=1  SampleTime=Ts
  Delay2 : Delay  DelayLength=1  SampleTime=Ts
  Gain2 : Gain  Gain=Ts
  Gain4 : Gain  Gain=Ts
  Gain6 : Gain  Gain=Ki_q
  Gain7 : Gain  Gain=Kp_q
  Gain8 : Gain  Gain=Ki_d
  Gain9 : Gain  Gain=Kp_d
  Sum2 : Sum  Inputs=++|
  Sum3 : Sum  Inputs=|++
  Sum4 : Sum  Inputs=-+|
  Sum5 : Sum  Inputs=|+-
  Sum6 : Sum  Inputs=|++
  Sum7 : Sum  Inputs=|++
  Vqe : Outport
  Vde : Outport  Port=2
  wires:
  Sum3/1 -> Vde/1  "Vde"
  Id_c/1 -> Sum5/1
  Sum2/1 -> Vqe/1  "Vqe"
  Iq/1 -> Sum4/1
  Gain6/1 -> Gain2/1
  Sum4/1 -> Gain7/1
  Sum6/1 -> Delay1/1, Sum2/2
  Iq_c/1 -> Sum4/2
  Id/1 -> Sum5/2
  Gain7/1 -> Sum2/1, Gain6/1
  Sum5/1 -> Gain9/1
  Gain9/1 -> Sum3/2, Gain8/1
  Gain2/1 -> Sum6/1
  Delay1/1 -> Sum6/2
  Gain4/1 -> Sum7/1
  Delay2/1 -> Sum7/2
  Sum7/1 -> Sum3/1, Delay2/1
  Gain8/1 -> Gain4/1

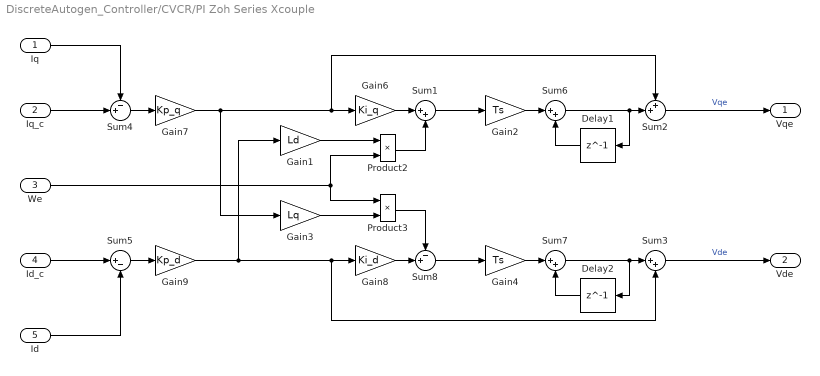
== system DiscreteAutogen_Controller/CVCR/PI Zoh Series Xcouple ==
  Iq : Inport
  Iq_c : Inport  Port=2
  We : Inport  Port=3
  Id_c : Inport  Port=4
  Id : Inport  Port=5
  Delay1 : Delay  DelayLength=1  SampleTime=Ts
  Delay2 : Delay  DelayLength=1  SampleTime=Ts
  Gain1 : Gain  Gain=Ld
  Gain2 : Gain  Gain=Ts
  Gain3 : Gain  Gain=Lq
  Gain4 : Gain  Gain=Ts
  Gain6 : Gain  Gain=Ki_q
  Gain7 : Gain  Gain=Kp_q
  Gain8 : Gain  Gain=Ki_d
  Gain9 : Gain  Gain=Kp_d
  Product2 : Product
  Product3 : Product
  Sum{1,3,6..7} (4 alike) : Sum  Inputs=|++
  Sum2 : Sum  Inputs=++|
  Sum4 : Sum  Inputs=-+|
  Sum5 : Sum  Inputs=|+-
  Sum8 : Sum  Inputs=-+|
  Vqe : Outport
  Vde : Outport  Port=2
  wires:
  Sum3/1 -> Vde/1  "Vde"
  Id_c/1 -> Sum5/1
  Sum2/1 -> Vqe/1  "Vqe"
  Iq/1 -> Sum4/1
  Gain6/1 -> Sum1/1
  Sum6/1 -> Delay1/1, Sum2/2
  Iq_c/1 -> Sum4/2
  Id/1 -> Sum5/2
  Gain7/1 -> Gain3/1, Sum2/1, Gain6/1
  Gain9/1 -> Gain1/1, Sum3/2, Gain8/1
  Gain2/1 -> Sum6/1
  Delay1/1 -> Sum6/2
  Gain4/1 -> Sum7/1
  Delay2/1 -> Sum7/2
  Sum7/1 -> Sum3/1, Delay2/1
  Sum4/1 -> Gain7/1
  Product3/1 -> Sum8/1
  Sum5/1 -> Gain9/1
  Product2/1 -> Sum1/2
  Sum1/1 -> Gain2/1
  Gain8/1 -> Sum8/2
  Sum8/1 -> Gain4/1
  We/1 -> Product2/2, Product3/1
  Gain1/1 -> Product2/1
  Gain3/1 -> Product3/2

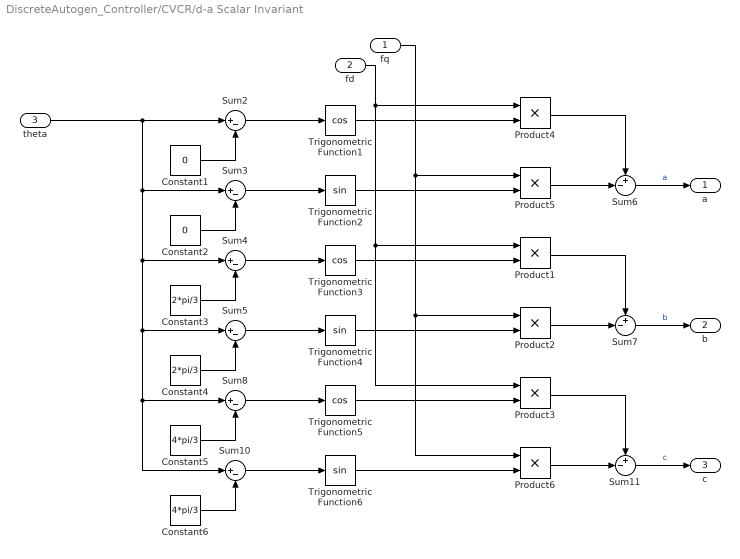
== system DiscreteAutogen_Controller/CVCR/d-a Scalar Invariant ==
  fq : Inport
  fd : Inport  Port=2
  theta : Inport  Port=3
  Constant1 : Constant  Value=0
  Constant2 : Constant  Value=0
  Constant3 : Constant  Value=2*pi/3
  Constant4 : Constant  Value=2*pi/3
  Constant5 : Constant  Value=4*pi/3
  Constant6 : Constant  Value=4*pi/3
  Product{1..6} (6 alike) : Product
  Sum{2..5,8,10} (6 alike) : Sum  Inputs=|+-
  Sum11 : Sum  Inputs=+-|
  Sum6 : Sum  Inputs=+-|
  Sum7 : Sum  Inputs=+-|
  Trigonometric Function1 : Trigonometry  Operator=cos
  Trigonometric Function2 : Trigonometry
  Trigonometric Function3 : Trigonometry  Operator=cos
  Trigonometric Function4 : Trigonometry
  Trigonometric Function5 : Trigonometry  Operator=cos
  Trigonometric Function6 : Trigonometry
  a : Outport
  b : Outport  Port=2
  c : Outport  Port=3
  wires:
  theta/1 -> Sum2/1, Sum3/1, Sum4/1, Sum5/1, Sum8/1, Sum10/1
  Trigonometric Function6/1 -> Product6/2
  Trigonometric Function5/1 -> Product3/2
  Constant4/1 -> Sum5/2
  Product1/1 -> Sum7/1
  Trigonometric Function1/1 -> Product4/2
  Product6/1 -> Sum11/2
  Sum10/1 -> Trigonometric Function6/1
  fd/1 -> Product3/1, Product1/1, Product4/1
  Sum3/1 -> Trigonometric Function2/1
  fq/1 -> Product6/1, Product2/1, Product5/1
  Product5/1 -> Sum6/2
  Trigonometric Function2/1 -> Product5/2
  Constant6/1 -> Sum10/2
  Sum8/1 -> Trigonometric Function5/1
  Sum2/1 -> Trigonometric Function1/1
  Sum4/1 -> Trigonometric Function3/1
  Constant1/1 -> Sum2/2
  Product2/1 -> Sum7/2
  Trigonometric Function3/1 -> Product1/2
  Sum5/1 -> Trigonometric Function4/1
  Trigonometric Function4/1 -> Product2/2
  Constant5/1 -> Sum8/2
  Sum6/1 -> a/1  "a"
  Constant3/1 -> Sum4/2
  Product3/1 -> Sum11/1
  Product4/1 -> Sum6/1
  Constant2/1 -> Sum3/2
  Sum11/1 -> c/1  "c"
  Sum7/1 -> b/1  "b"

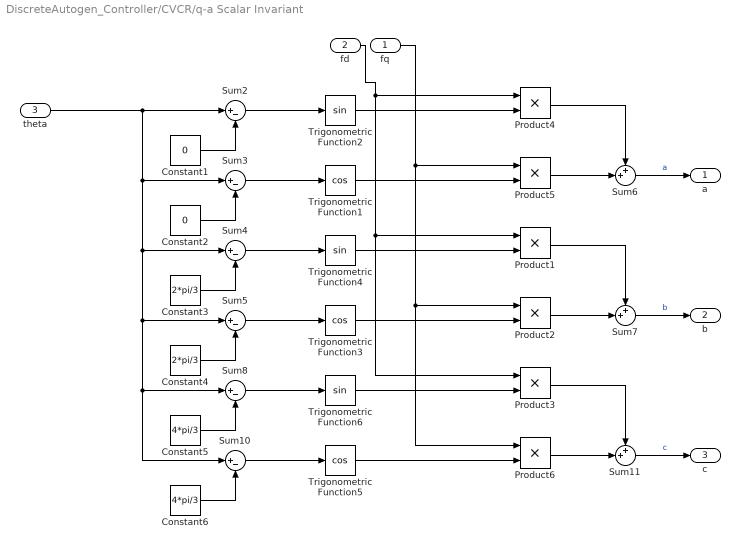
== system DiscreteAutogen_Controller/CVCR/q-a Scalar Invariant ==
  fq : Inport
  fd : Inport  Port=2
  theta : Inport  Port=3
  Constant1 : Constant  Value=0
  Constant2 : Constant  Value=0
  Constant3 : Constant  Value=2*pi/3
  Constant4 : Constant  Value=2*pi/3
  Constant5 : Constant  Value=4*pi/3
  Constant6 : Constant  Value=4*pi/3
  Product{1..6} (6 alike) : Product
  Sum{2..5,8,10} (6 alike) : Sum  Inputs=|+-
  Sum11 : Sum  Inputs=++|
  Sum6 : Sum  Inputs=++|
  Sum7 : Sum  Inputs=++|
  Trigonometric Function1 : Trigonometry  Operator=cos
  Trigonometric Function2 : Trigonometry
  Trigonometric Function3 : Trigonometry  Operator=cos
  Trigonometric Function4 : Trigonometry
  Trigonometric Function5 : Trigonometry  Operator=cos
  Trigonometric Function6 : Trigonometry
  a : Outport
  b : Outport  Port=2
  c : Outport  Port=3
  wires:
  Sum7/1 -> b/1  "b"
  Sum11/1 -> c/1  "c"
  Constant2/1 -> Sum3/2
  Product4/1 -> Sum6/1
  Product3/1 -> Sum11/1
  Constant3/1 -> Sum4/2
  Sum6/1 -> a/1  "a"
  Constant5/1 -> Sum8/2
  Trigonometric Function3/1 -> Product2/2
  Sum5/1 -> Trigonometric Function3/1
  Trigonometric Function4/1 -> Product1/2
  Product2/1 -> Sum7/2
  Constant1/1 -> Sum2/2
  Sum4/1 -> Trigonometric Function4/1
  Sum2/1 -> Trigonometric Function2/1
  Sum8/1 -> Trigonometric Function6/1
  Constant6/1 -> Sum10/2
  Trigonometric Function1/1 -> Product5/2
  Product5/1 -> Sum6/2
  fq/1 -> Product5/1, Product2/1, Product6/1
  Sum3/1 -> Trigonometric Function1/1
  fd/1 -> Product4/1, Product1/1, Product3/1
  Sum10/1 -> Trigonometric Function5/1
  Product6/1 -> Sum11/2
  Trigonometric Function2/1 -> Product4/2
  Product1/1 -> Sum7/1
  Constant4/1 -> Sum5/2
  Trigonometric Function6/1 -> Product3/2
  Trigonometric Function5/1 -> Product6/2
  theta/1 -> Sum10/1, Sum8/1, Sum5/1, Sum4/1, Sum3/1, Sum2/1

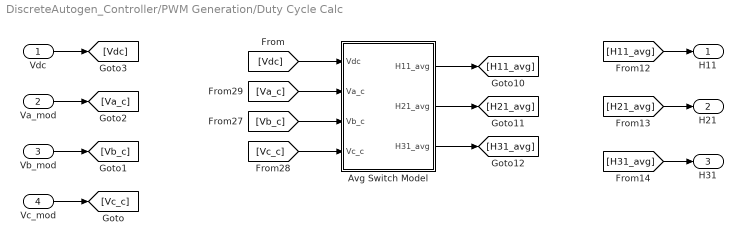
== system DiscreteAutogen_Controller/PWM Generation/Duty Cycle Calc ==
  Vdc : Inport
  Va_mod : Inport  Port=2
  Vb_mod : Inport  Port=3
  Vc_mod : Inport  Port=4
  Avg Switch Model : Subsystem
  H11 : Outport
  H21 : Outport  Port=2
  H31 : Outport  Port=3
  wires:
  Vdc/1 -> [Vdc]
  Vb_mod/1 -> [Vb_c]
  Va_mod/1 -> [Va_c]
  Vc_mod/1 -> [Vc_c]
  Avg Switch Model/3(H31_avg) -> [H31_avg]
  Avg Switch Model/2(H21_avg) -> [H21_avg]
  Avg Switch Model/1(H11_avg) -> [H11_avg]
  [Vc_c] -> Avg Switch Model/4(Vc_c)
  [Vb_c] -> Avg Switch Model/3(Vb_c)
  [Va_c] -> Avg Switch Model/2(Va_c)
  [Vdc] -> Avg Switch Model/1(Vdc)
  [H11_avg] -> H11/1
  [H21_avg] -> H21/1
  [H31_avg] -> H31/1

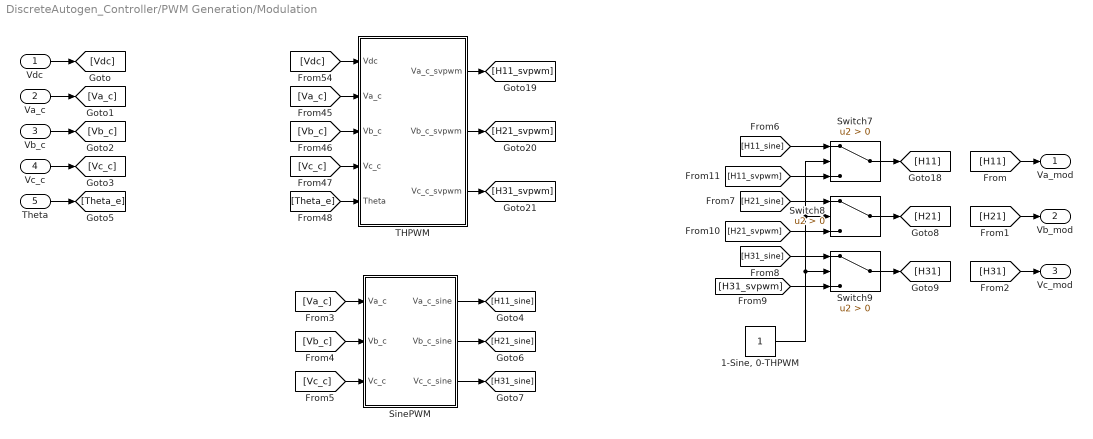
== system DiscreteAutogen_Controller/PWM Generation/Modulation ==
  Vdc : Inport
  Va_c : Inport  Port=2
  Vb_c : Inport  Port=3
  Vc_c : Inport  Port=4
  Theta : Inport  Port=5
  "1-Sine, 0-THPWM" : Constant
  SinePWM : Subsystem
  Switch7 : Switch  Criteria=u2 > Threshold  ZeroCross=off  SaturateOnIntegerOverflow=off  InputSameDT=off
  Switch8 : Switch  Criteria=u2 > Threshold  ZeroCross=off  SaturateOnIntegerOverflow=off  InputSameDT=off
  Switch9 : Switch  Criteria=u2 > Threshold  ZeroCross=off  SaturateOnIntegerOverflow=off  InputSameDT=off
  THPWM : Subsystem
  Va_mod : Outport
  Vb_mod : Outport  Port=2
  Vc_mod : Outport  Port=3
  wires:
  [Vc_c] -> SinePWM/3(Vc_c)
  [Va_c] -> SinePWM/1(Va_c)
  [Vb_c] -> SinePWM/2(Vb_c)
  SinePWM/3(Vc_c_sine) -> [H31_sine]
  SinePWM/2(Vb_c_sine) -> [H21_sine]
  SinePWM/1(Va_c_sine) -> [H11_sine]
  Switch8/1 -> [H21]
  [H31_sine] -> Switch9/1
  "1-Sine, 0-THPWM"/1 -> Switch7/2, Switch8/2, Switch9/2
  [H31_svpwm] -> Switch9/3
  Switch7/1 -> [H11]
  [H11_sine] -> Switch7/1
  [H21_svpwm] -> Switch8/3
  [H11_svpwm] -> Switch7/3
  Switch9/1 -> [H31]
  [H21_sine] -> Switch8/1
  [H31] -> Vc_mod/1
  [H21] -> Vb_mod/1
  [H11] -> Va_mod/1
  THPWM/3(Vc_c_svpwm) -> [H31_svpwm]
  THPWM/2(Vb_c_svpwm) -> [H21_svpwm]
  THPWM/1(Va_c_svpwm) -> [H11_svpwm]
  [Theta_e] -> THPWM/5(Theta)
  [Vc_c] -> THPWM/4(Vc_c)
  [Vb_c] -> THPWM/3(Vb_c)
  [Va_c] -> THPWM/2(Va_c)
  [Vdc] -> THPWM/1(Vdc)
  Theta/1 -> [Theta_e]
  Vc_c/1 -> [Vc_c]
  Vb_c/1 -> [Vb_c]
  Va_c/1 -> [Va_c]
  Vdc/1 -> [Vdc]

== system DiscreteAutogen_Controller/PWM Generation/Duty Cycle Calc/Avg Switch Model ==
  Vdc : Inport
  Va_c : Inport  Port=2
  Vb_c : Inport  Port=3
  Vc_c : Inport  Port=4
  Constant2 : Constant  Value=2
  Constant6 : Constant  Value=0
  Constant7 : Constant
  Divide{4..7} (4 alike) : Product  Inputs=/*
  Saturation Dynamic : simulink/Discontinuities/Saturation Dynamic  OutMin=[]  OutMax=[]  OutDataTypeStr=Inherit: Same as second input  OutDataType=fixdt(1, 16)  OutScaling=2^-10  DoSatur=off
  Saturation Dynamic1 : simulink/Discontinuities/Saturation Dynamic  OutMin=[]  OutMax=[]  OutDataTypeStr=Inherit: Same as second input  OutDataType=fixdt(1, 16)  OutScaling=2^-10  DoSatur=off
  Saturation Dynamic2 : simulink/Discontinuities/Saturation Dynamic  OutMin=[]  OutMax=[]  OutDataTypeStr=Inherit: Same as second input  OutDataType=fixdt(1, 16)  OutScaling=2^-10  DoSatur=off
  Sum1 : Sum  Inputs=++|
  Sum4 : Sum  Inputs=++|
  Sum5 : Sum  Inputs=++|
  H11_avg : Outport
  H21_avg : Outport  Port=2
  H31_avg : Outport  Port=3
  wires:
  Saturation Dynamic1/1 -> H21_avg/1
  Saturation Dynamic/1 -> H11_avg/1
  Vb_c/1 -> Sum4/2
  Vc_c/1 -> Sum1/2
  Vdc/1 -> Divide5/2, Divide4/1, Divide6/1, Divide7/1
  Va_c/1 -> Sum5/2
  Sum5/1 -> Divide4/2
  Divide7/1 -> Saturation Dynamic2/2
  Saturation Dynamic2/1 -> H31_avg/1
  Sum1/1 -> Divide7/2
  Divide6/1 -> Saturation Dynamic1/2
  Divide4/1 -> Saturation Dynamic/2
  Sum4/1 -> Divide6/2
  Constant6/1 -> Saturation Dynamic/3, Saturation Dynamic1/3, Saturation Dynamic2/3
  Constant2/1 -> Divide5/1
  Constant7/1 -> Saturation Dynamic2/1, Saturation Dynamic1/1, Saturation Dynamic/1
  Divide5/1 -> Sum5/1, Sum4/1, Sum1/1

== system DiscreteAutogen_Controller/PWM Generation/Modulation/SinePWM ==
  Va_c : Inport
  Vb_c : Inport  Port=2
  Vc_c : Inport  Port=3
  Va_c_sine : Outport
  Vb_c_sine : Outport  Port=2
  Vc_c_sine : Outport  Port=3
  wires:
  [H31_sine] -> Vc_c_sine/1
  [H21_sine] -> Vb_c_sine/1
  Vc_c/1 -> [Vc_c]
  Vb_c/1 -> [Vb_c]
  [H11_sine] -> Va_c_sine/1
  Va_c/1 -> [Va_c]
  [Va_c] -> [H11_sine]
  [Vb_c] -> [H21_sine]
  [Vc_c] -> [H31_sine]

== system DiscreteAutogen_Controller/PWM Generation/Modulation/THPWM ==
  Vdc : Inport
  Va_c : Inport  Port=2
  Vb_c : Inport  Port=3
  Vc_c : Inport  Port=4
  Theta : Inport  Port=5
  Constant1 : Constant  Value=pi/6
  Constant3 : Constant  Value=9
  Divide : Product  Inputs=*/
  Divide1 : Product  Inputs=**
  Gain1 : Gain  Gain=3
  Sum{1..4} (4 alike) : Sum  Inputs=|+-
  Trigonometric Function6 : Trigonometry
  Va_c_svpwm : Outport
  Vb_c_svpwm : Outport  Port=2
  Vc_c_svpwm : Outport  Port=3
  wires:
  Constant1/1 -> Sum4/2
  Sum4/1 -> Trigonometric Function6/1
  Divide1/1 -> Sum3/2, Sum2/2, Sum1/2  "zero_seq"
  Trigonometric Function6/1 -> Divide1/2
  Divide/1 -> Divide1/1
  Constant3/1 -> Divide/2
  Vdc/1 -> Divide/1
  Gain1/1 -> Sum4/1
  Theta/1 -> Gain1/1
  Sum2/1 -> Va_c_svpwm/1
  Sum3/1 -> Vc_c_svpwm/1
  Va_c/1 -> Sum2/1
  Vc_c/1 -> Sum3/1
  Sum1/1 -> Vb_c_svpwm/1
  Vb_c/1 -> Sum1/1
